simulink model "saturatedcontrol_with_integral_control101"  (R2024a)
settings: Solver=VariableStepAuto  StartTime=0.0  StopTime=20  RelTol=1e-3
undefined symbols (not defined in the file or in its folder): umax, umin
libraries: cstblocks x1
settings Model: Creator=barsr  LastModifiedBy=Anthony Rossiter
settings RTWCC: GPUComputeCapability=3.5

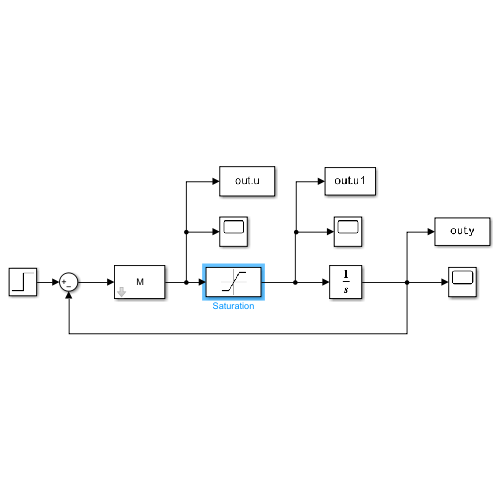
[thumbnail: Simulink's stored preview of the top-level diagram]
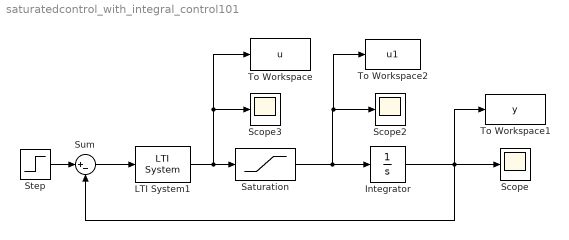
== system saturatedcontrol_with_integral_control101 ==
  Integrator : Integrator
  LTI System1 : cstblocks/LTI System  sys=M  IC=[]  PadeOrder=0
  Saturation : Saturate  UpperLimit=umax  LowerLimit=umin
  Scope : Scope
  Scope2 : Scope
  Scope3 : Scope
  Step : Step  Time=0  After=4  SampleTime=0
  Sum : Sum  Inputs=|+-
  To Workspace : ToWorkspace  VariableName=u  SaveFormat=Structure With Time  SampleTime=-1
  To Workspace1 : ToWorkspace  VariableName=y  SaveFormat=Structure With Time  SampleTime=-1
  To Workspace2 : ToWorkspace  VariableName=u1  SaveFormat=Structure With Time  SampleTime=-1
  wires:
  Step/1 -> Sum/1
  Saturation/1 -> Integrator/1, To Workspace2/1, Scope2/1
  Integrator/1 -> Scope/1, To Workspace1/1, Sum/2
  Sum/1 -> LTI System1/1
  LTI System1/1 -> To Workspace/1, Scope3/1, Saturation/1
